simulink model "maneuvering"  (R2016b)
settings: Solver=VariableStepAuto  StartTime=0.0  StopTime=200  RelTol=1e-3
undefined symbols (not defined in the file or in its folder): slcm
undefined symbols (not defined in the file): Hoerner, vessel, vesselABC
libraries: marine_gnc x1, marine_hydro x1
settings Model: Creator=Eier  LastModifiedBy=Eier

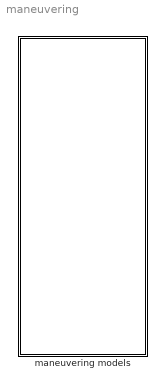
== system maneuvering ==
  maneuvering models : Subsystem

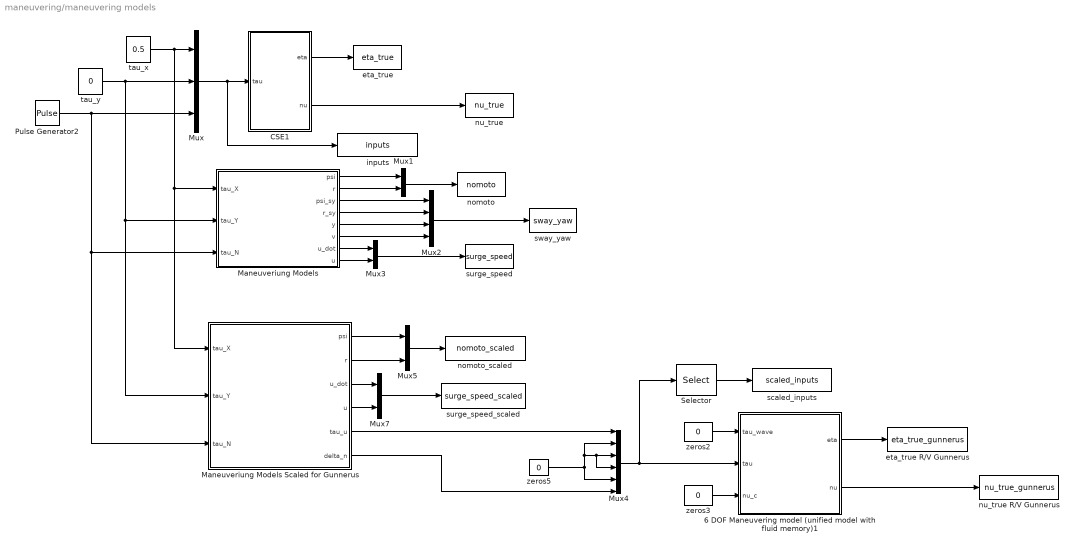
== system maneuvering/maneuvering models ==
  6 DOF Maneuvering model (unified model with fluid memory)1 : Subsystem  AncestorBlock=|  mask(ShipX (Veres) 6 DOF unified DP and maneuvering model){ABC=vesselABC, rho=1025, Axc=0.9*vessel.main.T*vessel.main.B, Ayc=0.9*vessel.main.T*vessel.main.Lpp, CX=1, CY_2D=Hoerner(vessel.main.B,vessel.main.T), Bv=vessel.Bv, Dp=vesselABC.Dp}
      | marine_hydro/Hydro Library/6 DOF Maneuvering model
      |  (unified model with fluid memory)
      mask prompts: ABC "Structure containing the fluid memory effects"; rho "Density of water (kg/m3)"; Axc "Frontal projected current area (m2)"; Ayc "Lateral projected current area (m2)"; CX "Current (drag) coefficient in surge CX"; CY_2D "2D drag coefficient in sway CY_2D"; Bv "Linear viscous damping matrix"; Dp "Linear potential damping"
      mask help:
      | System block containing the Shipx (Veres) 6 DOF unified DP and maneuvering model. The  6 DOF equations of motion also includes fluid memory effetcs. The data structure:
      |
      |    ABC.*           (>> load ABC )
      |
      | is generated using the Matlab script:
      |
      |    >> veres2ABC.m
      |
      | This script computes the retardation functions using state-space model approximations. It is also possible to include frequency-dependent viscous effects my editing the script.
      |
      | Author: Thor I. Fossen
      | -------------------------------------------------------------------------------------------------------------------------------------------------------
      | Reference:
      | T. I. Fossen and Ø. Smogeli (2004). Nonlinear Time-Domain Strip Theory Formulation for Low-Speed Maneuvering and Station-Keeping, Modelling, Identification and Control, MIC-25 (4):201-221.
      |
      | T. I. Fossen. A Nonlinear Unified State-Space Model for Ship Maneuvering and Control in a Seaway.  Journal of Bifurcation and Chaos (ENOC'05 Plenary), 2005.
  CSE1 : Subsystem
  Maneuveriung Models : Subsystem
  Maneuveriung Models Scaled for Gunnerus : Subsystem
  Mux : Mux  Inputs=3
  Mux{1,3,5,7} (4 alike) : Mux  Inputs=2
  Mux2 : Mux
  Mux4 : Mux  Inputs=6
  Pulse Generator2 : DiscretePulseGenerator  PulseType=Time based  Period=200  PulseWidth=10
  Selector : Selector  InputPortWidth=6  IndexOptions=Index vector (dialog)  Indices=[1 2 6]  OutputSizes=1
  eta_true : ToWorkspace  VariableName=eta_true  SaveFormat=Structure With Time  SampleTime=-1
  eta_true R/V Gunnerus : ToWorkspace  VariableName=eta_true_gunnerus  SaveFormat=Structure With Time  SampleTime=-1
  inputs : ToWorkspace  VariableName=inputs  SaveFormat=Structure With Time  SampleTime=-1
  nomoto : ToWorkspace  VariableName=nomoto  SaveFormat=Structure With Time  SampleTime=-1
  nomoto_scaled : ToWorkspace  VariableName=nomoto_scaled  SaveFormat=Structure With Time  SampleTime=-1
  nu_true : ToWorkspace  VariableName=nu_true  SaveFormat=Structure With Time  SampleTime=-1
  nu_true R/V Gunnerus : ToWorkspace  VariableName=nu_true_gunnerus  SaveFormat=Structure With Time  SampleTime=-1
  scaled_inputs : ToWorkspace  VariableName=scaled_inputs  SaveFormat=Structure With Time  SampleTime=-1
  surge_speed : ToWorkspace  VariableName=surge_speed  SaveFormat=Structure With Time  SampleTime=-1
  surge_speed_scaled : ToWorkspace  VariableName=surge_speed_scaled  SaveFormat=Structure With Time  SampleTime=-1
  sway_yaw : ToWorkspace  VariableName=sway_yaw  SaveFormat=Structure With Time  SampleTime=-1
  tau_x : Constant  Value=0.5
  tau_y : Constant  Value=0
  zeros2 : Constant  Value=0
  zeros3 : Constant  Value=0
  zeros5 : Constant  Value=0
  wires:
  Mux/1 -> inputs/1, CSE1/1(tau)
  Pulse Generator2/1 -> Maneuveriung Models Scaled for Gunnerus/3(tau_N), Maneuveriung Models/3(tau_N), Mux/3
  CSE1/1(eta) -> eta_true/1
  Maneuveriung Models/2(r) -> Mux1/2
  Mux1/1 -> nomoto/1
  Maneuveriung Models/6(v) -> Mux2/4
  Maneuveriung Models/4(r_sy) -> Mux2/2
  Maneuveriung Models/5(y) -> Mux2/3
  tau_x/1 -> Maneuveriung Models Scaled for Gunnerus/1(tau_X), Maneuveriung Models/1(tau_X), Mux/1
  tau_y/1 -> Maneuveriung Models/2(tau_Y), Maneuveriung Models Scaled for Gunnerus/2(tau_Y), Mux/2
  Maneuveriung Models/1(psi) -> Mux1/1
  Maneuveriung Models/3(psi_sy) -> Mux2/1
  Maneuveriung Models/7(u_dot) -> Mux3/1
  Maneuveriung Models/8(u) -> Mux3/2
  Mux3/1 -> surge_speed/1
  Mux4/1 -> Selector/1, 6 DOF Maneuvering model (unified model with fluid memory)1/2(tau)
  zeros5/1 -> Mux4/2, Mux4/3, Mux4/4, Mux4/5
  zeros2/1 -> 6 DOF Maneuvering model (unified model with fluid memory)1/1(tau_wave)
  zeros3/1 -> 6 DOF Maneuvering model (unified model with fluid memory)1/3(nu_c)
  Maneuveriung Models Scaled for Gunnerus/1(psi) -> Mux5/1
  Maneuveriung Models Scaled for Gunnerus/2(r) -> Mux5/2
  Mux7/1 -> surge_speed_scaled/1
  Maneuveriung Models Scaled for Gunnerus/3(u_dot) -> Mux7/1
  Maneuveriung Models Scaled for Gunnerus/4(u) -> Mux7/2
  Selector/1 -> scaled_inputs/1
  CSE1/2(nu) -> nu_true/1
  6 DOF Maneuvering model (unified model with fluid memory)1/2(nu) -> nu_true R/V Gunnerus/1
  6 DOF Maneuvering model (unified model with fluid memory)1/1(eta) -> eta_true R/V Gunnerus/1
  Maneuveriung Models Scaled for Gunnerus/5(tau_u) -> Mux4/1
  Mux5/1 -> nomoto_scaled/1
  Mux2/1 -> sway_yaw/1
  Maneuveriung Models Scaled for Gunnerus/6(delta_n) -> Mux4/6

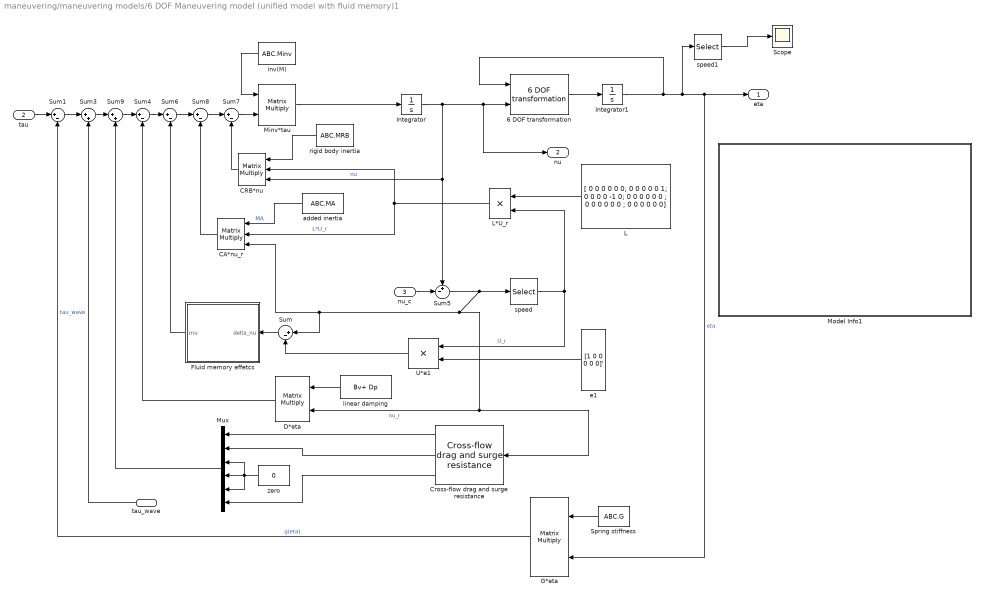
== system maneuvering/maneuvering models/6 DOF Maneuvering model (unified model with fluid memory)1 ==
  tau_wave : Inport
  tau : Inport  Port=2
  nu_c : Inport  Port=3
  6 DOF transformation : marine_gnc/Models/ Kinematics/6 DOF transformation
  CA*nu_r : Product  Inputs=3  Multiplication=Matrix(*)  RndMeth=Zero
  CRB*nu : Product  Inputs=3  Multiplication=Matrix(*)  RndMeth=Zero
  Cross-flow drag and surge resistance : marine_hydro/Hydro Library/Cross-flow drag and surge resistance  N=20  Lpp=vessel.main.Lpp  CD=CY_2D  Cx=CX  Ax=Axc  Ay=Ayc  rho_w=rho
  "D*eta " : Product  Multiplication=Matrix(*)  SaturateOnIntegerOverflow=on  OutDataTypeStr=Inherit: Same as first input
  Fluid memory effetcs : Subsystem
  G*eta : Product  Multiplication=Matrix(*)  SaturateOnIntegerOverflow=on  OutDataTypeStr=Inherit: Same as first input
  Integrator : Integrator
  Integrator1 : Integrator
  L : Constant  Value=|
      | [ 0     0     0     0     0     0;   0     0     0     0     0     1;
      |      0     0     0     0    -1     0;	
      |      0     0     0     0     0     0	;
      |      0     0     0     0     0     0	
      | ;     0     0     0     0     0     0]
  L*U_r : Product  RndMeth=Zero
  Minv*tau : Product  Inputs=**  Multiplication=Matrix(*)  SaturateOnIntegerOverflow=on  OutDataTypeStr=Inherit: Same as first input
  Model Info1 : Subsystem  LoadFcn=slcm LoadBlock;  InitFcn=slcm('UpdateAllCMBlocksInThisModelInit')  mask(CMBlock){InitialSaveTempField=, InitialBlockCM=, BlockCM=, Frame=on, SaveTempField=, DisplayStringWithTags=|, MaskDisplayString=This is an example block based on Perez and Fossen (2007).\nThe model includes speed-dependent fluid memory effects \ncross-flow drag and surge resistance (quadratic drag).\nYou must inlcude maneuvering coefficients your self. \n\nAlso notice that viscous roll damping is computed under the assumption \nof zero speed. Forward speed effects can, however, be added if necessary.\n\nReference\nT. Perez and T. I. Fossen (2007). Kinematic Models for Seakeeping\nand Maneuvering of Marine Vessels. Modeling, Identification\nand Control, MIC-28(1):1-12.\n\nDownload link: www.marinecontrol.org\n\nAuthor: Thor I. Fossen\n17-jul-2017 19:26:31, HorizontalTextAlignment=Left, LeftAlignmentValue=0.02, SourceBlockDiagram=maneuvering, TagMaxNumber=20, CMTag1=, CMTag2=, CMTag3=, CMTag4=, CMTag5=, CMTag6=, CMTag7=, CMTag8=, CMTag9=, CMTag10=, CMTag11=, CMTag12=, CMTag13=, CMTag14=, CMTag15=, CMTag16=, CMTag17=, CMTag18=, CMTag19=, CMTag20=}
      mask DisplayStringWithTags=|
      | This is an example block based on Perez and Fossen (2007).\nThe model includes speed-dependent fluid memory effects
      | cross-flow drag and surge resistance (quadratic drag).\nYou must inlcude maneuvering coefficients your self. \n
      | Also notice that viscous roll damping is computed under the assumption \nof zero speed. Forward speed effects can, however, be added if necessary.
      |
      | Reference
      | T. Perez and T. I. Fossen (2007). Kinematic Models for Seakeeping
      | and Maneuvering of Marine Vessels. Modeling, Identification\nand Control, MIC-28(1):1-12.\n
      | Download link: www.marinecontrol.org
      |
      | Author: Thor I. Fossen
      | %<LastModificationDate>
      mask help: This block allows revision control information to be displayed within the model.
      settings: CopyFcn=slcm CopyBlock;  DeleteFcn=slcm Cancel;  PostSaveFcn=slcm('UpdateAllCMBlocksInThisModel')  NameChangeFcn=slcm Rename;  OpenFcn=slcm
      mask Display: text(str2num(LeftAlignmentValue), 0.5, MaskDisplayString, 'HorizontalAlignment', HorizontalTextAlignment)
  Mux : Mux  Inputs=6
  Scope : Scope
  Spring stiffness : Constant  Value=ABC.G
  Sum : Sum  Inputs=|+-
  Sum{1,4,6..8} (5 alike) : Sum  Inputs=|+-  SaturateOnIntegerOverflow=on
  Sum3 : Sum  Inputs=|++  SaturateOnIntegerOverflow=on
  Sum5 : Sum  Inputs=+-|  SaturateOnIntegerOverflow=on
  Sum9 : Sum  Inputs=|++  SaturateOnIntegerOverflow=on
  U*e1 : Product  RndMeth=Zero
  added inertia : Constant  Value=ABC.MA
  e1 : Constant  Value=[1 0 0 0 0 0]'  VectorParams1D=off
  inv(M) : Constant  Value=ABC.Minv
  linear damping : Constant  Value=Bv+ Dp
  rigid body inertia : Constant  Value=ABC.MRB
  speed : Selector  InputPortWidth=6  IndexOptions=Index vector (dialog)  Indices=[1]  OutputSizes=1
  speed1 : Selector  InputPortWidth=6  IndexOptions=Index vector (dialog)  Indices=[6]  OutputSizes=1
  zero : Constant  Value=0
  eta : Outport
  nu : Outport  Port=2
  wires:
  Minv*tau/1 -> Integrator/1
  Sum4/1 -> Sum6/1
  Sum6/1 -> Sum8/1
  Sum3/1 -> Sum9/1
  tau_wave/1 -> Sum3/2  "tau_wave"
  tau/1 -> Sum1/1
  rigid body inertia/1 -> CRB*nu/1
  G*eta/1 -> Sum1/2  "g(eta)"
  Integrator1/1 -> speed1/1, eta/1, G*eta/2, 6 DOF transformation/1  "eta"
  6 DOF transformation/1 -> Integrator1/1
  added inertia/1 -> CA*nu_r/1  "MA"
  Spring stiffness/1 -> G*eta/1
  Sum1/1 -> Sum3/1
  Integrator/1 -> 6 DOF transformation/2, nu/1, Sum5/1, CRB*nu/3  "nu"
  linear damping/1 -> "D*eta "/1
  "D*eta "/1 -> Sum4/2
  nu_c/1 -> Sum5/2
  Sum5/1 -> "D*eta "/2, Cross-flow drag and surge resistance/1, CA*nu_r/3, Sum/1, speed/1  "nu_r"
  Sum7/1 -> Minv*tau/2
  Fluid memory effetcs/1(mu) -> Sum6/2
  CRB*nu/1 -> Sum7/2
  Sum8/1 -> Sum7/1
  CA*nu_r/1 -> Sum8/2
  Cross-flow drag and surge resistance/1 -> Mux/1
  Cross-flow drag and surge resistance/2 -> Mux/2
  Cross-flow drag and surge resistance/3 -> Mux/6
  zero/1 -> Mux/4, Mux/3, Mux/5
  Sum9/1 -> Sum4/1
  Mux/1 -> Sum9/2
  L/1 -> L*U_r/1
  L*U_r/1 -> CRB*nu/2, CA*nu_r/2  "L*U_r"
  Sum/1 -> Fluid memory effetcs/1(delta_nu)
  U*e1/1 -> Sum/2
  e1/1 -> U*e1/2
  inv(M)/1 -> Minv*tau/1
  speed/1 -> U*e1/1, L*U_r/2  "U_r"
  speed1/1 -> Scope/1

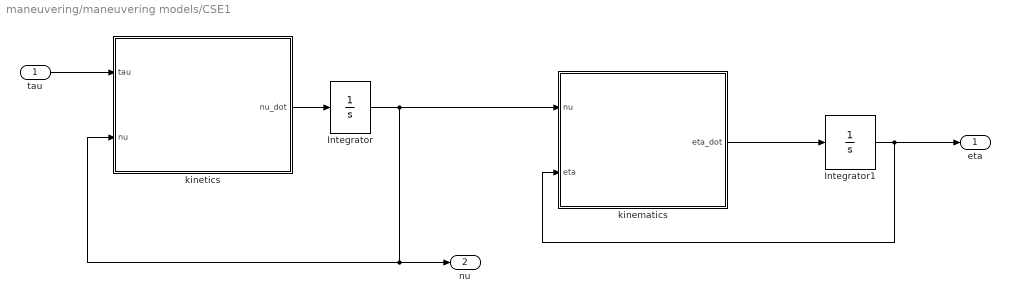
== system maneuvering/maneuvering models/CSE1 ==
  tau : Inport
  Integrator : Integrator  InitialCondition=[0 0 0]'
  Integrator1 : Integrator  InitialCondition=[0 0 0]'
  kinematics : MATLAB Function  TreatAsAtomicUnit=on
  kinetics : MATLAB Function  TreatAsAtomicUnit=on
  eta : Outport
  nu : Outport  Port=2
  wires:
  kinetics/1(nu_dot) -> Integrator/1
  Integrator1/1 -> eta/1, kinematics/2(eta)
  kinematics/1(eta_dot) -> Integrator1/1
  tau/1 -> kinetics/1(tau)
  Integrator/1 -> kinematics/1(nu), kinetics/2(nu), nu/1

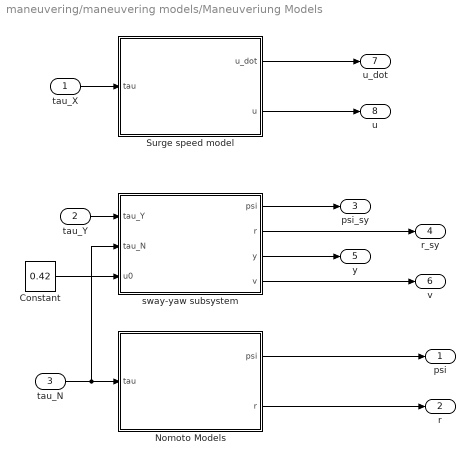
== system maneuvering/maneuvering models/Maneuveriung Models ==
  tau_X : Inport
  tau_Y : Inport  Port=2
  tau_N : Inport  Port=3
  Constant : Constant  Value=0.42
  Nomoto Models : Subsystem
  Surge speed model : Subsystem
  sway-yaw subsystem : Subsystem
  psi : Outport
  r : Outport  Port=2
  psi_sy : Outport  Port=3
  r_sy : Outport  Port=4
  y : Outport  Port=5
  v : Outport  Port=6
  u_dot : Outport  Port=7
  u : Outport  Port=8
  wires:
  tau_N/1 -> Nomoto Models/1(tau), sway-yaw subsystem/2(tau_N)
  Nomoto Models/1(psi) -> psi/1
  Nomoto Models/2(r) -> r/1
  tau_Y/1 -> sway-yaw subsystem/1(tau_Y)
  sway-yaw subsystem/2(r) -> r_sy/1
  sway-yaw subsystem/3(y) -> y/1
  sway-yaw subsystem/4(v) -> v/1
  sway-yaw subsystem/1(psi) -> psi_sy/1
  tau_X/1 -> Surge speed model/1(tau)
  Surge speed model/1(u_dot) -> u_dot/1
  Surge speed model/2(u) -> u/1
  Constant/1 -> sway-yaw subsystem/3(u0)

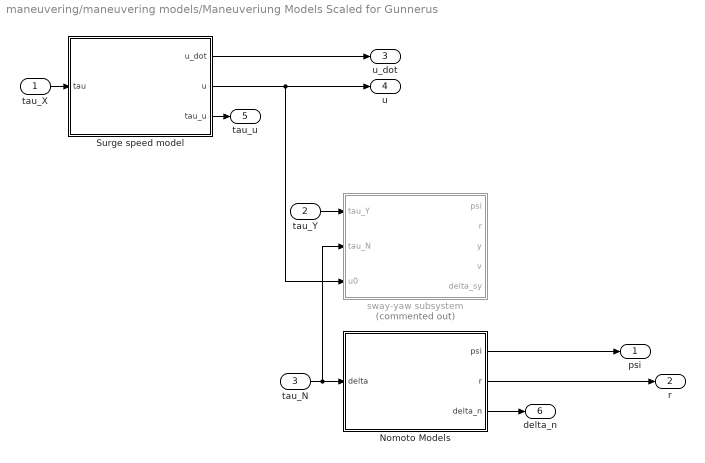
== system maneuvering/maneuvering models/Maneuveriung Models Scaled for Gunnerus ==
  tau_X : Inport
  tau_Y : Inport  Port=2
  tau_N : Inport  Port=3
  Nomoto Models : Subsystem
  Surge speed model : Subsystem
  sway-yaw subsystem : Subsystem  Commented=on
  psi : Outport
  r : Outport  Port=2
  u_dot : Outport  Port=3
  u : Outport  Port=4
  tau_u : Outport  Port=5
  delta_n : Outport  Port=6
  wires:
  tau_N/1 -> sway-yaw subsystem/2(tau_N), Nomoto Models/1(delta)
  Nomoto Models/1(psi) -> psi/1
  Nomoto Models/2(r) -> r/1
  tau_Y/1 -> sway-yaw subsystem/1(tau_Y)
  tau_X/1 -> Surge speed model/1(tau)
  Surge speed model/1(u_dot) -> u_dot/1
  Surge speed model/2(u) -> sway-yaw subsystem/3(u0), u/1
  Surge speed model/3(tau_u) -> tau_u/1
  Nomoto Models/3(delta_n) -> delta_n/1

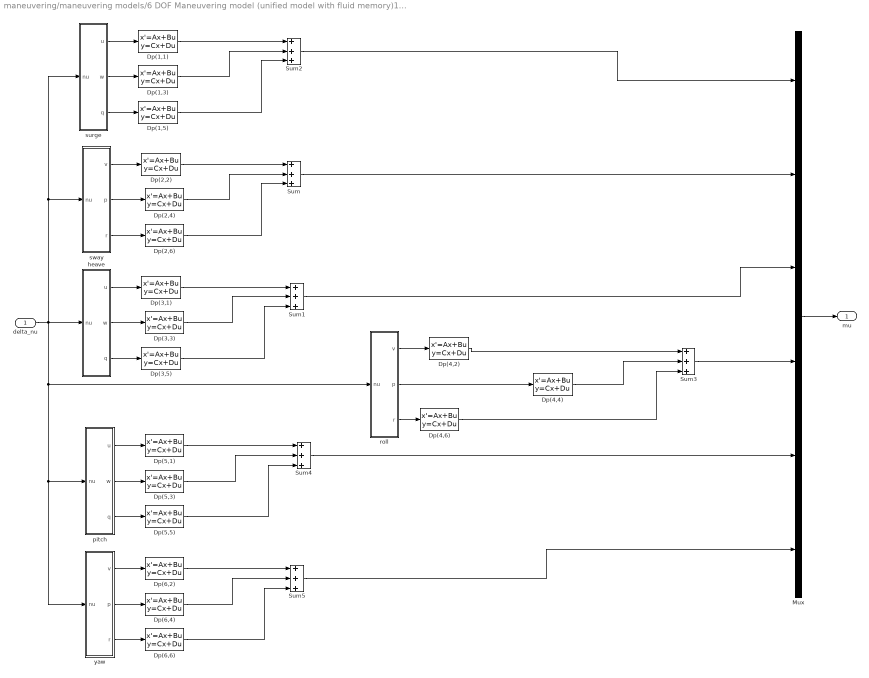
== system maneuvering/maneuvering models/6 DOF Maneuvering model (unified model with fluid memory)1/Fluid memory effetcs ==
  delta_nu : Inport
  Dp(1,1) : StateSpace  A=ABC.Ar{1,1}  B=ABC.Br{1,1}  C=ABC.Cr{1,1}  D=ABC.Dr{1,1}  X0=0
  Dp(1,3) : StateSpace  A=ABC.Ar{1,3}  B=ABC.Br{1,3}  C=ABC.Cr{1,3}  D=ABC.Dr{1,3}  X0=0
  Dp(1,5) : StateSpace  A=ABC.Ar{1,5}  B=ABC.Br{1,5}  C=ABC.Cr{1,5}  D=ABC.Dr{1,5}  X0=0
  Dp(2,2) : StateSpace  A=ABC.Ar{2,2}  B=ABC.Br{2,2}  C=ABC.Cr{2,2}  D=ABC.Dr{2,2}  X0=0
  Dp(2,4) : StateSpace  A=ABC.Ar{2,4}  B=ABC.Br{2,4}  C=ABC.Cr{2,4}  D=ABC.Dr{2,4}  X0=0
  Dp(2,6) : StateSpace  A=ABC.Ar{2,6}  B=ABC.Br{2,6}  C=ABC.Cr{2,6}  D=ABC.Dr{2,6}  X0=0
  Dp(3,1) : StateSpace  A=ABC.Ar{3,1}  B=ABC.Br{3,1}  C=ABC.Cr{3,1}  D=ABC.Dr{3,1}  X0=0
  Dp(3,3) : StateSpace  A=ABC.Ar{3,3}  B=ABC.Br{3,3}  C=ABC.Cr{3,3}  D=ABC.Dr{3,3}  X0=0
  Dp(3,5) : StateSpace  A=ABC.Ar{3,5}  B=ABC.Br{3,5}  C=ABC.Cr{3,5}  D=ABC.Dr{3,5}  X0=0
  Dp(4,2) : StateSpace  A=ABC.Ar{4,2}  B=ABC.Br{4,2}  C=ABC.Cr{4,2}  D=ABC.Dr{4,2}  X0=0
  Dp(4,4) : StateSpace  A=ABC.Ar{4,4}  B=ABC.Br{4,4}  C=ABC.Cr{4,4}  D=ABC.Dr{4,4}  X0=0
  Dp(4,6) : StateSpace  A=ABC.Ar{4,6}  B=ABC.Br{4,6}  C=ABC.Cr{4,6}  D=ABC.Dr{4,6}  X0=0
  Dp(5,1) : StateSpace  A=ABC.Ar{5,1}  B=ABC.Br{5,1}  C=ABC.Cr{5,1}  D=ABC.Dr{5,1}  X0=0
  Dp(5,3) : StateSpace  A=ABC.Ar{5,3}  B=ABC.Br{5,3}  C=ABC.Cr{5,3}  D=ABC.Dr{5,3}  X0=0
  Dp(5,5) : StateSpace  A=ABC.Ar{5,5}  B=ABC.Br{5,5}  C=ABC.Cr{5,5}  D=ABC.Dr{5,5}  X0=0
  Dp(6,2) : StateSpace  A=ABC.Ar{6,2}  B=ABC.Br{6,2}  C=ABC.Cr{6,2}  D=ABC.Dr{6,2}  X0=0
  Dp(6,4) : StateSpace  A=ABC.Ar{6,4}  B=ABC.Br{6,4}  C=ABC.Cr{6,4}  D=ABC.Dr{6,4}  X0=0
  Dp(6,6) : StateSpace  A=ABC.Ar{6,6}  B=ABC.Br{6,6}  C=ABC.Cr{6,6}  D=ABC.Dr{6,6}  X0=0
  Mux : Mux  Inputs=6
  Sum{,1..5} (6 alike) : Sum  Inputs=+++  SaturateOnIntegerOverflow=on
  heave : Subsystem
  pitch : Subsystem
  roll : Subsystem
  surge : Subsystem
  sway : Subsystem
  yaw : Subsystem
  mu : Outport
  wires:
  Dp(4,4)/1 -> Sum3/2
  roll/2(p) -> Dp(4,4)/1
  Sum5/1 -> Mux/6
  yaw/3(r) -> Dp(6,6)/1
  yaw/2(p) -> Dp(6,4)/1
  yaw/1(v) -> Dp(6,2)/1
  Dp(6,6)/1 -> Sum5/3
  Dp(6,4)/1 -> Sum5/2
  Dp(6,2)/1 -> Sum5/1
  Sum3/1 -> Mux/4
  Dp(5,1)/1 -> Sum4/1
  pitch/1(u) -> Dp(5,1)/1
  pitch/2(w) -> Dp(5,3)/1
  pitch/3(q) -> Dp(5,5)/1
  Dp(5,5)/1 -> Sum4/3
  Dp(5,3)/1 -> Sum4/2
  roll/3(r) -> Dp(4,6)/1
  roll/1(v) -> Dp(4,2)/1
  Dp(4,6)/1 -> Sum3/3
  Dp(4,2)/1 -> Sum3/1
  Dp(1,1)/1 -> Sum2/1
  surge/1(u) -> Dp(1,1)/1
  surge/2(w) -> Dp(1,3)/1
  surge/3(q) -> Dp(1,5)/1
  Sum2/1 -> Mux/1
  Dp(1,5)/1 -> Sum2/3
  Dp(1,3)/1 -> Sum2/2
  Mux/1 -> mu/1
  delta_nu/1 -> yaw/1(nu), pitch/1(nu), roll/1(nu), surge/1(nu), sway/1(nu), heave/1(nu)
  Dp(3,1)/1 -> Sum1/1
  heave/1(u) -> Dp(3,1)/1
  heave/2(w) -> Dp(3,3)/1
  heave/3(q) -> Dp(3,5)/1
  Sum1/1 -> Mux/3
  Dp(3,5)/1 -> Sum1/3
  Dp(3,3)/1 -> Sum1/2
  sway/3(r) -> Dp(2,6)/1
  sway/2(p) -> Dp(2,4)/1
  sway/1(v) -> Dp(2,2)/1
  Sum/1 -> Mux/2
  Dp(2,6)/1 -> Sum/3
  Dp(2,4)/1 -> Sum/2
  Dp(2,2)/1 -> Sum/1
  Sum4/1 -> Mux/5

== system maneuvering/maneuvering models/6 DOF Maneuvering model (unified model with fluid memory)1/Model Info1 ==
  EmptySubsystem : Subsystem

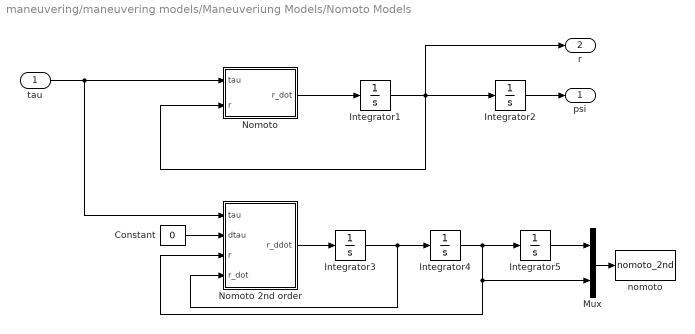
== system maneuvering/maneuvering models/Maneuveriung Models/Nomoto Models ==
  tau : Inport
  Constant : Constant  Value=0
  Integrator{1..5} (5 alike) : Integrator
  Mux : Mux  Inputs=2
  Nomoto : MATLAB Function  TreatAsAtomicUnit=on
  Nomoto 2nd order : MATLAB Function  TreatAsAtomicUnit=on
  nomoto : ToWorkspace  VariableName=nomoto_2nd  SaveFormat=Structure With Time  SampleTime=-1
  psi : Outport
  r : Outport  Port=2
  wires:
  Nomoto/1(r_dot) -> Integrator1/1
  Integrator1/1 -> r/1, Integrator2/1, Nomoto/2(r)
  Integrator2/1 -> psi/1
  Nomoto 2nd order/1(r_ddot) -> Integrator3/1
  Integrator3/1 -> Integrator4/1, Nomoto 2nd order/4(r_dot)
  Integrator4/1 -> Integrator5/1, Nomoto 2nd order/3(r), Mux/2
  tau/1 -> Nomoto 2nd order/1(tau), Nomoto/1(tau)
  Constant/1 -> Nomoto 2nd order/2(dtau)
  Integrator5/1 -> Mux/1
  Mux/1 -> nomoto/1

== system maneuvering/maneuvering models/Maneuveriung Models/Surge speed model ==
  tau : Inport
  " Surge Speed Model" : MATLAB Function  TreatAsAtomicUnit=on
  Integrator : Integrator
  u_dot : Outport
  u : Outport  Port=2
  wires:
  " Surge Speed Model"/1(u_dot) -> Integrator/1, u_dot/1
  tau/1 -> " Surge Speed Model"/1(tau)
  Integrator/1 -> " Surge Speed Model"/2(nu), u/1

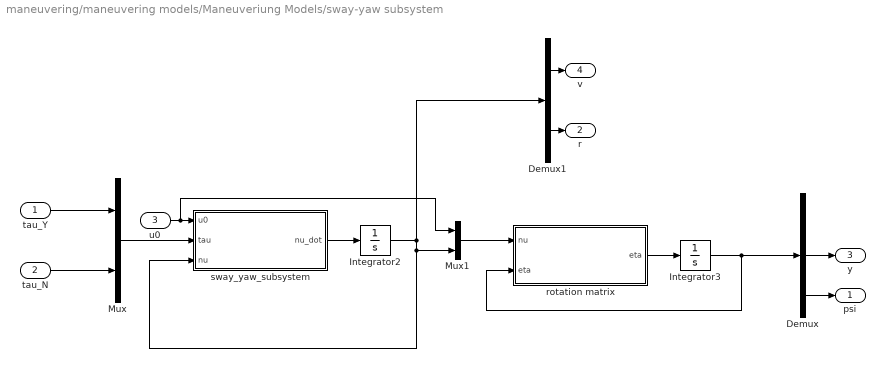
== system maneuvering/maneuvering models/Maneuveriung Models/sway-yaw subsystem ==
  tau_Y : Inport
  tau_N : Inport  Port=2
  u0 : Inport  Port=3
  Demux : Demux  Outputs=3
  Demux1 : Demux  Outputs=2
  Integrator2 : Integrator  InitialCondition=[0 0]'
  Integrator3 : Integrator  InitialCondition=[0 0 0]'
  Mux : Mux  Inputs=2
  Mux1 : Mux  Inputs=2
  rotation matrix : MATLAB Function  TreatAsAtomicUnit=on
  sway_yaw_subsystem : MATLAB Function  TreatAsAtomicUnit=on
  psi : Outport
  r : Outport  Port=2
  y : Outport  Port=3
  v : Outport  Port=4
  wires:
  tau_N/1 -> Mux/2
  tau_Y/1 -> Mux/1
  Mux/1 -> sway_yaw_subsystem/2(tau)
  sway_yaw_subsystem/1(nu_dot) -> Integrator2/1
  Integrator2/1 -> Mux1/2, sway_yaw_subsystem/3(nu), Demux1/1
  u0/1 -> Mux1/1, sway_yaw_subsystem/1(u0)
  rotation matrix/1(eta) -> Integrator3/1
  Integrator3/1 -> Demux/1, rotation matrix/2("eta ")
  Demux1/2 -> r/1
  Demux1/1 -> v/1
  Mux1/1 -> rotation matrix/1(nu)
  Demux/3 -> psi/1
  Demux/2 -> y/1

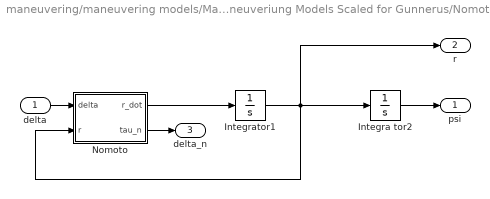
== system maneuvering/maneuvering models/Maneuveriung Models Scaled for Gunnerus/Nomoto Models ==
  delta : Inport
  Integra tor2 : Integrator
  Integrator1 : Integrator
  Nomoto : MATLAB Function  TreatAsAtomicUnit=on
  psi : Outport
  r : Outport  Port=2
  delta_n : Outport  Port=3
  wires:
  Integrator1/1 -> r/1, Integra tor2/1, Nomoto/2(r)
  Integra tor2/1 -> psi/1
  delta/1 -> Nomoto/1(delta)
  Nomoto/2(tau_n) -> delta_n/1
  Nomoto/1(r_dot) -> Integrator1/1

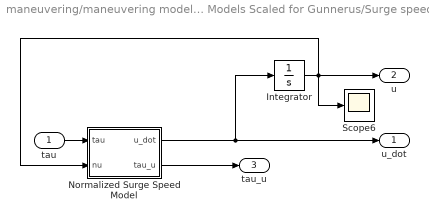
== system maneuvering/maneuvering models/Maneuveriung Models Scaled for Gunnerus/Surge speed model ==
  tau : Inport
  Integrator : Integrator
  Normalized Surge Speed Model : MATLAB Function  TreatAsAtomicUnit=on
  Scope6 : Scope
  u_dot : Outport
  u : Outport  Port=2
  tau_u : Outport  Port=3
  wires:
  Normalized Surge Speed Model/1(u_dot) -> Integrator/1, u_dot/1
  Integrator/1 -> Scope6/1, u/1, Normalized Surge Speed Model/2(nu)
  tau/1 -> Normalized Surge Speed Model/1(tau)
  Normalized Surge Speed Model/2(tau_u) -> tau_u/1

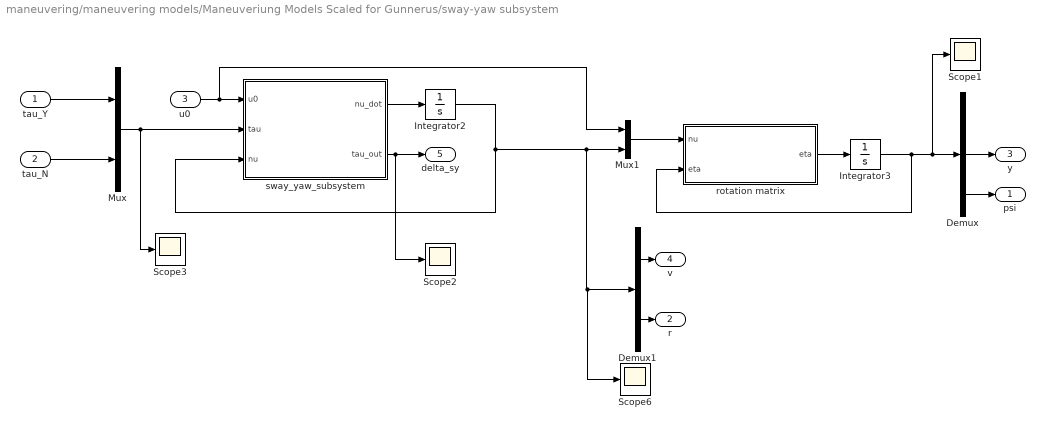
== system maneuvering/maneuvering models/Maneuveriung Models Scaled for Gunnerus/sway-yaw subsystem ==
  tau_Y : Inport
  tau_N : Inport  Port=2
  u0 : Inport  Port=3
  Demux : Demux  Outputs=3
  Demux1 : Demux  Outputs=2
  Integrator2 : Integrator  InitialCondition=[0 0]'
  Integrator3 : Integrator  InitialCondition=[0 0 0]'
  Mux : Mux  Inputs=2
  Mux1 : Mux  Inputs=2
  Scope{1..3,6} (4 alike) : Scope
  rotation matrix : MATLAB Function  TreatAsAtomicUnit=on
  sway_yaw_subsystem : MATLAB Function  TreatAsAtomicUnit=on
  psi : Outport
  r : Outport  Port=2
  y : Outport  Port=3
  v : Outport  Port=4
  delta_sy : Outport  Port=5
  wires:
  tau_N/1 -> Mux/2
  tau_Y/1 -> Mux/1
  Mux/1 -> Scope3/1, sway_yaw_subsystem/2(tau)
  sway_yaw_subsystem/1(nu_dot) -> Integrator2/1
  u0/1 -> sway_yaw_subsystem/1(u0), Mux1/1
  sway_yaw_subsystem/2(tau_out) -> Scope2/1, delta_sy/1
  Integrator2/1 -> Scope6/1, Demux1/1, Mux1/2, sway_yaw_subsystem/3(nu)
  rotation matrix/1(eta) -> Integrator3/1
  Integrator3/1 -> Scope1/1, Demux/1, rotation matrix/2("eta ")
  Demux1/2 -> r/1
  Demux1/1 -> v/1
  Mux1/1 -> rotation matrix/1(nu)
  Demux/3 -> psi/1
  Demux/2 -> y/1

== system maneuvering/maneuvering models/6 DOF Maneuvering model (unified model with fluid memory)1/Fluid memory effetcs/heave ==
  nu : Inport
  Selector : Selector  InputPortWidth=6  IndexOptions=Index vector (dialog)  Indices=[1]  OutputSizes=1
  Selector1 : Selector  InputPortWidth=6  IndexOptions=Index vector (dialog)  Indices=[3]  OutputSizes=1
  Selector2 : Selector  InputPortWidth=6  IndexOptions=Index vector (dialog)  Indices=[5]  OutputSizes=1
  u : Outport
  w : Outport  Port=2
  q : Outport  Port=3
  wires:
  Selector2/1 -> q/1
  Selector1/1 -> w/1
  Selector/1 -> u/1
  nu/1 -> Selector2/1, Selector1/1, Selector/1

== system maneuvering/maneuvering models/6 DOF Maneuvering model (unified model with fluid memory)1/Fluid memory effetcs/pitch ==
  nu : Inport
  Selector : Selector  InputPortWidth=6  IndexOptions=Index vector (dialog)  Indices=[1]  OutputSizes=1
  Selector1 : Selector  InputPortWidth=6  IndexOptions=Index vector (dialog)  Indices=[3]  OutputSizes=1
  Selector2 : Selector  InputPortWidth=6  IndexOptions=Index vector (dialog)  Indices=[5]  OutputSizes=1
  u : Outport
  w : Outport  Port=2
  q : Outport  Port=3
  wires:
  Selector2/1 -> q/1
  Selector1/1 -> w/1
  Selector/1 -> u/1
  nu/1 -> Selector2/1, Selector1/1, Selector/1

== system maneuvering/maneuvering models/6 DOF Maneuvering model (unified model with fluid memory)1/Fluid memory effetcs/roll ==
  nu : Inport
  Selector : Selector  InputPortWidth=6  IndexOptions=Index vector (dialog)  Indices=[2]  OutputSizes=1
  Selector1 : Selector  InputPortWidth=6  IndexOptions=Index vector (dialog)  Indices=[4]  OutputSizes=1
  Selector2 : Selector  InputPortWidth=6  IndexOptions=Index vector (dialog)  Indices=[6]  OutputSizes=1
  v : Outport
  p : Outport  Port=2
  r : Outport  Port=3
  wires:
  Selector2/1 -> r/1
  Selector1/1 -> p/1
  Selector/1 -> v/1
  nu/1 -> Selector2/1, Selector1/1, Selector/1

== system maneuvering/maneuvering models/6 DOF Maneuvering model (unified model with fluid memory)1/Fluid memory effetcs/surge ==
  nu : Inport
  Selector : Selector  InputPortWidth=6  IndexOptions=Index vector (dialog)  Indices=[1]  OutputSizes=1
  Selector1 : Selector  InputPortWidth=6  IndexOptions=Index vector (dialog)  Indices=[3]  OutputSizes=1
  Selector2 : Selector  InputPortWidth=6  IndexOptions=Index vector (dialog)  Indices=[5]  OutputSizes=1
  u : Outport
  w : Outport  Port=2
  q : Outport  Port=3
  wires:
  Selector2/1 -> q/1
  Selector1/1 -> w/1
  Selector/1 -> u/1
  nu/1 -> Selector2/1, Selector1/1, Selector/1

== system maneuvering/maneuvering models/6 DOF Maneuvering model (unified model with fluid memory)1/Fluid memory effetcs/sway ==
  nu : Inport
  Selector : Selector  InputPortWidth=6  IndexOptions=Index vector (dialog)  Indices=[2]  OutputSizes=1
  Selector1 : Selector  InputPortWidth=6  IndexOptions=Index vector (dialog)  Indices=[4]  OutputSizes=1
  Selector2 : Selector  InputPortWidth=6  IndexOptions=Index vector (dialog)  Indices=[6]  OutputSizes=1
  v : Outport
  p : Outport  Port=2
  r : Outport  Port=3
  wires:
  Selector2/1 -> r/1
  Selector1/1 -> p/1
  Selector/1 -> v/1
  nu/1 -> Selector2/1, Selector1/1, Selector/1

== system maneuvering/maneuvering models/6 DOF Maneuvering model (unified model with fluid memory)1/Fluid memory effetcs/yaw ==
  nu : Inport
  Selector : Selector  InputPortWidth=6  IndexOptions=Index vector (dialog)  Indices=[2]  OutputSizes=1
  Selector1 : Selector  InputPortWidth=6  IndexOptions=Index vector (dialog)  Indices=[4]  OutputSizes=1
  Selector2 : Selector  InputPortWidth=6  IndexOptions=Index vector (dialog)  Indices=[6]  OutputSizes=1
  v : Outport
  p : Outport  Port=2
  r : Outport  Port=3
  wires:
  Selector2/1 -> r/1
  Selector1/1 -> p/1
  Selector/1 -> v/1
  nu/1 -> Selector2/1, Selector1/1, Selector/1

== system maneuvering/maneuvering models/6 DOF Maneuvering model (unified model with fluid memory)1/Model Info1/EmptySubsystem ==

== matlab function maneuvering/maneuvering models/Maneuveriung Models/sway-yaw subsystem/rotation matrix ==
  data: nu input; eta input; eta output
function eta = body2ned(nu,eta)
psi=eta(3);
R=[cos(psi) -sin(psi) 0;
    sin(psi) cos(psi) 0;
    0 0 1];

eta=R*nu;
end

== matlab function maneuvering/maneuvering models/Maneuveriung Models Scaled for Gunnerus/sway-yaw subsystem/rotation matrix ==
  data: nu input; eta input; eta output
function eta = body2ned(nu,eta)
psi=eta(3);
R=[cos(psi) -sin(psi) 0;
    sin(psi) cos(psi) 0;
    0 0 1];

eta=R*nu;
end

== matlab function maneuvering/maneuvering models/Maneuveriung Models/Surge speed model/ Surge Speed Model ==
  data: tau input; nu input; u_dot output
function u_dot  = fcn(tau,nu)
m    = 14.79;
g=9.81;
L=1;
u=nu(1);

X_ud  =     -2.0;
m_11 = m-X_ud;

X_u		= -0.6555;		
X_uu 	= 0.3545;	
X_uuu 	= -3.787;
d_11 = -X_u - X_uu*u-X_uuu*u^2;
M_bis=m_11/m;
D_bis=d_11/(m*sqrt(g/L));
tau_bis=tau/(m*g);

u_dot = 1/(m*M_bis)*(tau-m*sqrt(g/L)*D_bis*u);
end

== matlab function maneuvering/maneuvering models/Maneuveriung Models/Nomoto Models/Nomoto ==
  data: tau input; r input; r_dot output
function r_dot  = fcn(tau,r)
K=0.45;
T=2;

g=9.81;
L=1;

K_bis=1/sqrt(g/L)*K;
T_bis=1/sqrt(L/g)*T;

r_dot=-(sqrt(g/L)*1/T_bis)*r+g/L*(K_bis/T_bis)*tau;

end

== matlab function maneuvering/maneuvering models/Maneuveriung Models/sway-yaw subsystem/sway_yaw_subsystem ==
  data: u0 input; tau input; nu_dot output; nu input
function nu_dot = sway_yaw_subsystem(u0,tau, nu)
u = u0;
v   = nu(1);
r   = nu(2);

%% MATRICES

m    = 14.79;   I_z  =  1.7600;   x_g = 0.0375;       % x_g  =  0.0460; % Table B.1

g=9.81;
L=1;
%% Added mass
X_ud=-2.0;
Y_vd =     -1.0;	N_vd =    -0.0;		% Table B.1 guestimate
Y_rd =      -0.0;	N_rd =    -1.0;		% Table B.1

%% Total mass matrix
m_22 = m-Y_vd;
m_23 = m*x_g-Y_rd;
m_32 = m*x_g-N_vd;
m_33 = I_z-N_rd;

M    = [m_22 m_23;m_32 m_33];

%% Damping coefficients
% Comments at the end of the lines indicate the old values used.
Y_v		= -1.33; 			
Y_vv	= -2.776;			
Y_vvv	= -64.91;			
						
Y_rv	= -0.805;			

N_r		= -1.900; 
N_rr	= -0.750; 
N_rrr	= 0;
						
N_vr	= 0.080; 

%% Correolis matrix
c_23 = (m-X_ud)*u;
C = [0     c_23; (X_ud-Y_vd)*u (m*x_g-Y_rd)*u];

%% Assembly of the damping matrix
% d_22 = -Y_v - Y_vv*v - Y_vvv*v^2 - Y_rv*abs(r);
% d_33 = -N_r - N_rr*abs(r) - N_rrr*r^2 - N_vr*abs(v); % using abs(r)
d_22 = -Y_v;%- Y_vv*v - Y_vvv*v^2 - Y_rv*abs(r);
d_33 = -N_r;%- N_rr*abs(r) - N_rrr*r^2 - N_vr*abs(v); % using abs(r)
d_23 = 0;
d_32 = 0;

D    = [d_22 d_23;d_32 d_33];


%% CALCULATION

T=diag([1 1/L]);

M_bis=(T^(-1)*(T^(2)*M)*T)/m;
N_bis=(T^(-1)*(T^(2)*(D+C))*T)/(m*sqrt(g/L));
tau_bis=T*tau/(m*g);

%nu_dot = (m*T^(-2)*(T*M_bis*T^(-1)))\(m*g*T^(-1)*tau_bis-m*sqrt(g/L)*T^(-2)*(T*N_bis*T^(-1))*nu);

nu_dot = M\(tau-(C+D)*nu);

== matlab function maneuvering/maneuvering models/Maneuveriung Models/Nomoto Models/Nomoto 2nd order ==
  data: tau input; dtau input; r input; r_dot input; r_ddot output
function r_ddot  = fcn(tau,dtau,r,r_dot)
K=0.45;
T1=3;
T2=1;
T3=2;

g=9.81;
L=1;

K_bis=1/sqrt(g/L)*K;
T1_bis=1/sqrt(L/g)*T1;
T2_bis=1/sqrt(L/g)*T2;
T3_bis=1/sqrt(L/g)*T3;

c1=L/g*(T1_bis*T2_bis);
c2=sqrt(L/g)*(T1_bis+T2_bis);
c3=sqrt(g/L)*K_bis;

r_ddot=-c2/c1*r_dot-1/c1*r+c3/c1*(tau-T3_bis*dtau);

end

== matlab function maneuvering/maneuvering models/Maneuveriung Models Scaled for Gunnerus/Nomoto Models/Nomoto ==
  data: delta input; r input; r_dot output; tau_n output
function [r_dot,tau_n]  = fcn(delta,r)
K=0.45;
T=2;
m=14.79;
mG = 743888.94;
g=9.81;
L=1;
LG=28.9;

K_bis=1/sqrt(g/L)*K;
T_bis=1/sqrt(L/g)*T;
b=1e6;

r_dot=-sqrt(g/LG)/T_bis*r+g/LG*(K_bis/T_bis)*delta;

tau_n=b*delta;
end

== matlab function maneuvering/maneuvering models/Maneuveriung Models Scaled for Gunnerus/Surge speed model/Normalized Surge Speed Model ==
  data: tau input; nu input; u_dot output; tau_u output
function [u_dot,tau_u]  = fcn(tau,nu)
m=14.79;
mG    = 743888.94;
g=9.81;
L=1;
LG=29.8;
u=nu(1);
b=1;
delta=tau/b;
X_ud  = -2.0;
m_11 = m-X_ud;

X_u		= -0.6555;		
X_uu 	= 0.3545;	
X_uuu 	= -3.787;
d_11 = (-X_u - X_uu*u-X_uuu*u^2);
M_bis=m_11/m;
D_bis=d_11/(m*sqrt(g/L));
b_bis=tau/(m*g);
bG=2.5*b_bis*mG*g;

tau_u=bG*delta;

u_dot = (mG*M_bis)\(0.5*b_bis*mG*g*delta-mG*sqrt(g/LG)*D_bis*u);
end

== matlab function maneuvering/maneuvering models/Maneuveriung Models Scaled for Gunnerus/sway-yaw subsystem/sway_yaw_subsystem ==
  data: u0 input; tau input; nu_dot output; nu input; tau_out output size=2
function [nu_dot,tau_out] = sway_yaw_subsystem(u0,tau, nu)
u = u0;
v   = nu(1);
r   = nu(2);

%% MATRICES
m    = 14.79;   I_z  =  1.7600;   x_g = 0.0375;       % x_g  =  0.0460; % Table B.1


m=14.79;
mG = 743888.94;
g=9.81;
L=1;
LG=29.8;

%% Added mass
X_ud=-2.0;
Y_vd =     -1.0;	N_vd =    -0.0;		% Table B.1 guestimate
Y_rd =      -0.0;	N_rd =    -1.0;		% Table B.1

%% Total mass matrix
m_22 = m-Y_vd;
m_23 = m*x_g-Y_rd;
m_32 = m*x_g-N_vd;
m_33 = I_z-N_rd;

M    = [m_22 m_23;m_32 m_33];

%% Damping coefficients
% Comments at the end of the lines indicate the old values used.
Y_v		= -1.33; 			
Y_vv	= -2.776;			
Y_vvv	= -64.91;			
						
Y_rv	= -0.805;			

N_r		= -1.900; 
N_rr	= -0.750; 
						
N_vr	= 0.080; 

%% Correolis matrix
% c_23 =1/(sqrt(g*L))*(m-X_ud)*u;
% C = [0     c_23; (X_ud-Y_vd)*1/sqrt(g*L)*u (m*x_g-Y_rd)*1/sqrt(g*L)*u];

c_23 =(m-X_ud)*u;
C = [0     c_23; (X_ud-Y_vd)*u (m*x_g-Y_rd)*u];
%% Assembly of the damping matrix
d_22 = -Y_v;%-Y_vv*v - Y_vvv*v^2 - Y_rv*abs(r);
d_33 = -N_r;% - N_rr*abs(r) - N_vr*abs(v); % using abs(r)

d_23 = 0;
d_32 = 0;

D    = [d_22 d_23;d_32 d_33];

%% CALCULATION


T=diag([1 1/L]);
TG=diag([1 1/LG]);

M_bis=(T^(-1)*(T^(2)*M)*T)/m;
N_bis=(T^(-1)*(T^(2)*(D+C))*T)/(m*sqrt(g/L));
b=mG*LG/(m*L)*[0.67 0.67]';
delta=1;
tau_bis=[tau(1)/(m*g);tau(2)/(m*g*L)];
tau_mod=[tau_bis(1)*mG*g;tau_bis(2)*mG*g*LG];
tau_out=b.*tau;
nu_dot = (mG*TG^(-2)*(TG*M_bis*TG^(-1)))\(tau_out-mG*sqrt(g/LG)*TG^(-2)*(TG*N_bis*TG^(-1))*nu);

== matlab function maneuvering/maneuvering models/CSE1/kinematics ==
  data: nu input; eta_dot output; eta input
function eta_dot = CSE1_eta_dot(nu,eta)

psi = eta(3);

J = [cos(psi) -sin(psi) 0
     sin(psi) cos(psi)  0
     0        0         1];

eta_dot = J*nu;

== matlab function maneuvering/maneuvering models/CSE1/kinetics ==
  data: tau input; nu_dot output; nu input
function nu_dot = CSE1_nu_dot(tau,nu)

u   = nu(1);
v   = nu(2);
r   = nu(3);

%% MATRICES

m    = 14.79;   I_z  =  1.7600;   x_g = 0.0375;       % x_g  =  0.0460; % Table B.1


%% Added mass
X_ud  =     -2.0;											% Table B.1
					Y_vd =     -1.0;	N_vd =    -0.0;		% Table B.1 guestimate
					Y_rd =      -0.0;	N_rd =    -1.0;		% Table B.1

%% Total mass matrix
m_11 = m-X_ud;
m_22 = m-Y_vd;
m_23 = m*x_g-Y_rd;
m_32 = m*x_g-N_vd;
m_33 = I_z-N_rd;

M    = [m_11 0    0
        0    m_22 m_23
        0    m_32 m_33];
	
%% Damping coefficients
% Comments at the end of the lines indicate the old values used.
X_u		= -0.6555;		
X_uu 	= 0.3545;		
X_uuu 	= -3.787;		

Y_v		= -1.33; 			
Y_vv	= -2.776;			
Y_vvv	= -64.91;			
						
Y_rv	= -0.805;			

N_r		= -1.900; % N_r
N_rr	= -0.750; % N_rr
N_rrr	= 0;
						
N_vr	= 0.080; % N_rv, N_vr

%% Correolis matrix
c_13 = -(m-Y_vd)*v-(m*x_g-Y_rd)*r;
c_23 = (m-X_ud)*u;
C    = [0     0     c_13
        0     0     c_23
        -c_13 -c_23 0];

%% Assembly of the damping matrix
d_11 = -X_u - X_uu*u - X_uuu*u^2;
d_22 = -Y_v - Y_vv*v - Y_vvv*v^2 - Y_rv*abs(r);
d_33 = -N_r - N_rr*abs(r) - N_rrr*r^2 - N_vr*abs(v); % using abs(r)

D    = [d_11 0 0
        0    d_22 0
        0    0 d_33];


%% CALCULATION
nu_dot = M\(tau-(C+D)*nu);
